simulink model "drones_simulation"  (R2025b)
settings: Solver=ode4  StartTime=0.0  StopTime=t_sim  FixedStep=Ts  RelTol=1e-3
values from neighbouring files (symbols this model uses):
  adj_row_1 = Adj_mat(1,:)    [Parameters_scenarios.m]
  adj_row_2 = Adj_mat(2,:)    [Parameters_scenarios.m]
  adj_row_3 = Adj_mat(3,:)    [Parameters_scenarios.m]
  adj_row_4 = Adj_mat(4,:)    [Parameters_scenarios.m]
  gamma1 = 8.0    (= 8)    [Parameters_scenarios.m]
  gamma2 = 8.0    (= 8)    [Parameters_scenarios.m]
  goal_tolerance = 0.05    [Parameters_scenarios.m]
  Ib = diag([Jxx, Jyy, Jzz])    [Parameters_scenarios.m]
  Kd = 2.5    [Parameters_scenarios.m]
  Kp = 1.2    [Parameters_scenarios.m]
  mass = 0.032    [Parameters_scenarios.m]
  max_acc = 2.5    [Parameters_scenarios.m]
  max_vel = 1.2 * (dist_total / desired_flight_time)    [Parameters_scenarios.m]
  Rc = 2.0    (= 2)    [Parameters_scenarios.m]
  Rs = Rs_safe    (= 0.15)    [Parameters_scenarios.m]
  Rs_obs = radius_robots + radii_obstacles + margin    (= 0.95)    [Parameters_scenarios.m]
  v0_1 = v0(1,:)'    [Parameters_scenarios.m]
  v0_2 = v0(2,:)'    [Parameters_scenarios.m]
  v0_3 = v0(3,:)'    [Parameters_scenarios.m]
  v0_4 = v0(4,:)'    [Parameters_scenarios.m]
  x0_1 = x0(1,:)'    [Parameters_scenarios.m]
  x0_2 = x0(2,:)'    [Parameters_scenarios.m]
  x0_3 = x0(3,:)'    [Parameters_scenarios.m]
  x0_4 = x0(4,:)'    [Parameters_scenarios.m]
  x_objects = [0.0 ... (first row only)    [Parameters_scenarios.m]
  xg_1 = xg(1,:)'    [Parameters_scenarios.m]
  xg_2 = xg(2,:)'    [Parameters_scenarios.m]
  xg_3 = xg(3,:)'    [Parameters_scenarios.m]
  xg_4 = xg(4,:)'    [Parameters_scenarios.m]
  xg_vec = reshape(xg', [], 1)    [Parameters_scenarios.m]
libraries: robotcorelib x4
(part 2 of 3)

== matlab function drones_simulation/Safety_and_connectivity_Drone_4/MATLAB Function10 ==
  data: x_i input; v_i input; u_safe output; x_neighbors input; v_neighbors input; u_gtg input; gamma1 input; gamma2 input; Rs input; x_obs input; Rs_obs input; x_comm input; v_comm input; Rc input; max_acc input
function u_safe = QPsafety_i(x_i, v_i, x_neighbors, v_neighbors, u_gtg, ...
                             gamma1, gamma2, Rs, x_obs, Rs_obs, ...
                             x_comm, v_comm, Rc, max_acc)
%QPsafety_i  Filtra un comando nominale u_gtg con un QP + vincoli CBF/HOCBF.
%
% IDEA:
%   - Variabile ottimizzata: u (accelerazione 3D).
%   - Obiettivo: restare il più vicino possibile al comando nominale u_gtg.
%   - Vincoli: evitare ostacoli, evitare collisioni con vicini, mantenere connettività,
%              e non scendere sotto una quota minima (pavimento virtuale).
%
% FORMA QP (quadprog):
%   min_u   1/2 u' H u + f' u
%   s.t.    A u <= b -> vincoli per mantenere distanze e connettività
%           lb <= u <=  -> vincolo per non superare i limiti di
%           accelerazione
%
% 
%   I vincoli CBF usano una forma tipo "relative degree 2":
%       h_ddot + gamma1*h_dot + gamma2*h >= 0
%   che diventa un vincolo lineare in u (quindi compatibile con quadprog).

    %% (0) Dimensione del problema
    n_dims = 3;   % accelerazione 3D [ux; uy; uz]

    %% (1) Output di default
    % Se non serve filtrare o il QP non trova soluzione, almeno ritorniamo qualcosa.
    u_safe = u_gtg;

    %% (2) Constraints sull'accelerazione
    lb = -max_acc * ones(n_dims, 1);
    ub =  max_acc * ones(n_dims, 1);

    %% (3) Costo del QP: minimizza ||u - u_gtg||^2
    % quadprog minimizza: 1/2 u'Hu + f'u
    % Con H=2I e f=-2u_gtg, si ottiene (a costante vicina):
    %    1/2 u'(2I)u + (-2u_gtg)'u = u'u - 2u_gtg'u  ~ ||u-u_gtg||^2
    H_qp = 2 * eye(n_dims);
    f_qp = -2 * u_gtg;

    %% (4) Matrici vincoli lineari (si riempiono aggiungendo righe)
    % Ogni ostacolo/vicino genera un vincolo lineare del tipo: a^T u <= b
    A = zeros(0, n_dims);
    b = zeros(0, 1);

    %% (5) VINCOLI 1: Ostacoli statici (evitamento)
    % Barriera: h = ||p - p_obs||^2 - R^2 >= 0  (stai FUORI dalla sfera di raggio R)
    % Con doppio integratore: h_ddot = LfLfh + LgLfh*u
    % Vincolo HOCBF: h_ddot + gamma1*h_dot + gamma2*h >= 0
    n_obs = size(x_obs, 2);

    for k = 1:n_obs
        p_o = x_obs(:, k);      % posizione ostacolo k
        R_o = Rs_obs(k);        % raggio di sicurezza ostacolo k

        rel_p = x_i - p_o;      % posizione relativa
        rel_v = v_i;            % ostacolo fermo => v_rel = v_i

        dist_sq = norm(rel_p)^2;
        h      = dist_sq - R_o^2;
        h_dot  = 2 * rel_p' * rel_v;

        % Per h = ||rel_p||^2 - R^2:
        % LgLfh = 2*rel_p' (coefficiente davanti a u)
        % LfLfh = 2*||rel_v||^2 (termine noto, non dipende da u)
        LgLfh = 2 * rel_p';
        LfLfh = 2 * (rel_v' * rel_v);

        % quadprog vuole A*u <= b.
        % Dalla forma HOCBF si arriva a:  -(LgLfh) * u <= LfLfh + gamma1*h_dot + gamma2*h
        A = [A; -LgLfh];
        b = [b; (LfLfh + gamma1*h_dot + gamma2*h)];
    end

    %% (6) VINCOLI 2: Vicini (anti-collisione inter-agente)
    % Stesso tipo di barriera degli ostacoli, ma con posizione/velocità relative:
    %   h = ||p_i - p_j||^2 - Rs^2 >= 0  (distanza minima Rs)
    valid_cols = ~isnan(x_neighbors(1,:));
    n_max_neighbors = size(x_neighbors, 2);

    for k = 1:n_max_neighbors
        if valid_cols(k)
            p_j = x_neighbors(:, k);
            v_j = v_neighbors(:, k);

            rel_p = x_i - p_j;
            rel_v = v_i - v_j;

            dist_sq = norm(rel_p)^2;
            h      = dist_sq - Rs^2;
            h_dot  = 2 * rel_p' * rel_v;

            LgLfh = 2 * rel_p';
            LfLfh = 2 * (rel_v' * rel_v);

            A = [A; -LgLfh];
            b = [b; (LfLfh + gamma1*h_dot + gamma2*h)];
        end
    end

    %% (7) VINCOLI 3: Connettività / coesione (non allontanarsi oltre Rc)
    % Qui la barriera è "invertita" (stai DENTRO):
    %   h_c = Rc^2 - ||p_i - p_c||^2 >= 0  =>  ||p_i - p_c|| <= Rc
    valid_cols_comm = ~isnan(x_comm(1,:));
    n_max_comm = size(x_comm, 2);

    for k = 1:n_max_comm
        if valid_cols_comm(k)
            p_c = x_comm(:, k);
            v_c = v_comm(:, k);

            rel_p = x_i - p_c;
            rel_v = v_i - v_c;

            dist_sq = norm(rel_p)^2;

            h_c     = Rc^2 - dist_sq;
            h_dot_c = -2 * rel_p' * rel_v;

            % Segni diversi rispetto al caso "stai fuori":
            LgLfh_c = -2 * rel_p';
            LfLfh_c = -2 * (rel_v' * rel_v);

            % Anche qui si porta tutto in A*u <= b:
            A = [A; -LgLfh_c];
            b = [b; (LfLfh_c + gamma1*h_dot_c + gamma2*h_c)];
        end
    end

    %% (8) VINCOLO 4: Pavimento virtuale (z >= z_limit)
    % Barriera: h = z - z_limit >= 0
    % Con doppio integratore: h_dot = v_z, h_ddot = u_z
    z_limit = 0.1;

    z_pos = x_i(3);
    z_vel = v_i(3);

    h_floor     = z_pos - z_limit;
    h_dot_floor = z_vel;

    % Seleziona solo la componente u_z:
    LgLfh_floor = [0, 0, 1];
    LfLfh_floor = 0;

    % Vincolo: u_z + gamma1*v_z + gamma2*(z-z_limit) >= 0
    % => -u_z <= gamma1*v_z + gamma2*h_floor
    A = [A; -LgLfh_floor];   % [0 0 -1]
    b = [b; (LfLfh_floor + gamma1*h_dot_floor + gamma2*h_floor)];

    %% (9) Risoluzione del QP
    % Se non ci sono vincoli, restituisci direttamente u_gtg.
    if isempty(A)
        u_safe = u_gtg;
        return;
    end

    options = optimoptions('quadprog', ...
        'Algorithm', 'active-set', ...
        'Display', 'off');

    % Punto iniziale per il solver (warm start semplice)
    u0 = zeros(n_dims, 1);

    % Risolvi:
    [u_opt, ~, exitflag] = quadprog(H_qp, f_qp, A, b, [], [], lb, ub, u0, options);

    %% (10) Scelta finale dell'azione
    if exitflag == 1
        % Soluzione trovata: comando sicuro
        u_safe = u_opt;
    else
        % QP infeasible / non risolto: fallback conservativo (frenata)
        % u = -k*v riduce la velocità rapidamente
        u_safe = -2.0 * v_i;
    end
end

== matlab function drones_simulation/Safety_and_connectivity_Drone_3/MATLAB Function11 ==
  data: x_neighbors output; x_i input; x_all input; v_all input; Rs input; v_neighbors output
function [x_neighbors, v_neighbors] = select_neighbors_i(x_i, x_all, v_all, Rs)
%Funzione usata per selezionare i vicini entro un raggio Rs dal robot i.
%
% SCOPO:
%   Dato lo stato del robot corrente (posizione x_i) e lo stato di tutti i robot
%   (x_all, v_all impacchettati in un unico vettore), questa funzione:
%   - scorre tutti i robot j
%   - scarta se stesso
%   - calcola la distanza tra i e j
%   - se j è entro Rs, lo inserisce nella lista dei vicini.
%
% INPUT:
%   x_i   : [3x1] posizione del robot corrente (p_i)
%   x_all : [3N x 1] posizioni di tutti i robot impacchettate
%           (x1;y1;z1; x2;y2;z2; ... ; xN;yN;zN)
%   v_all : [3N x 1] velocità di tutti i robot impacchettate
%           (vx1;vy1;vz1; vx2;vy2;vz2; ... )
%   Rs    : raggio di sicurezza
%
% OUTPUT:
%   x_neighbors : [3 x (N-1)] posizioni dei robot vicini trovati
%   v_neighbors : [3 x (N-1)] velocità dei robot vicini trovati
%   (Le colonne non usate restano NaN.)

    %% Parametri base
    n_dims   = 3;                          % dimensione spazio (x,y,z)
    n_robots = length(x_all) / n_dims;     % numero totale di robot N

    %% Preallocazione output con nan
    x_neighbors = nan(n_dims, n_robots-1);
    v_neighbors = nan(n_dims, n_robots-1);

    %% Contatore vicini trovati e raggio al quadrato
    count = 0;
    r_sq  = Rs^2;

    %% Scorri tutti i robot e seleziona quelli entro Rs
    for j = 1:n_robots

        %si estrae posizione e velocità del robot j dal vettore
        %impacchettato - INDICI
        idx_start = (j-1)*n_dims + 1;
        idx_end   = j*n_dims;

        p_j = x_all(idx_start : idx_end);  % [3x1] posizione robot j
        v_j = v_all(idx_start : idx_end);  % [3x1] velocità robot j

        % Si esclude il robot corrente 
        if norm(x_i - p_j) < 1e-6
            continue;
        end

        % Calcola la distanza al quadrato tra robot i e robot j
        dist_sq = sum((x_i - p_j).^2);

        % Se il robot j è entro Rs, aggiungilo alla lista dei vicini
        if dist_sq <= r_sq
            count = count + 1;

            x_neighbors(:, count) = p_j;
            v_neighbors(:, count) = v_j;
        end
    end

    % Al termine:
    % - Le prime "count" colonne contengono i vicini effettivi.
    % - Le colonne restanti rimangono NaN.
end

== matlab function drones_simulation/Safety_and_connectivity_Drone_4/MATLAB Function12 ==
  data: x_neighbors output; x_i input; x_all input; v_all input; Rs input; v_neighbors output
function [x_neighbors, v_neighbors] = select_neighbors_i(x_i, x_all, v_all, Rs)
%Funzione usata per selezionare i vicini entro un raggio Rs dal robot i.
%
% SCOPO:
%   Dato lo stato del robot corrente (posizione x_i) e lo stato di tutti i robot
%   (x_all, v_all impacchettati in un unico vettore), questa funzione:
%   - scorre tutti i robot j
%   - scarta se stesso
%   - calcola la distanza tra i e j
%   - se j è entro Rs, lo inserisce nella lista dei vicini.
%
% INPUT:
%   x_i   : [3x1] posizione del robot corrente (p_i)
%   x_all : [3N x 1] posizioni di tutti i robot impacchettate
%           (x1;y1;z1; x2;y2;z2; ... ; xN;yN;zN)
%   v_all : [3N x 1] velocità di tutti i robot impacchettate
%           (vx1;vy1;vz1; vx2;vy2;vz2; ... )
%   Rs    : raggio di sicurezza
%
% OUTPUT:
%   x_neighbors : [3 x (N-1)] posizioni dei robot vicini trovati
%   v_neighbors : [3 x (N-1)] velocità dei robot vicini trovati
%   (Le colonne non usate restano NaN.)

    %% Parametri base
    n_dims   = 3;                          % dimensione spazio (x,y,z)
    n_robots = length(x_all) / n_dims;     % numero totale di robot N

    %% Preallocazione output con nan
    x_neighbors = nan(n_dims, n_robots-1);
    v_neighbors = nan(n_dims, n_robots-1);

    %% Contatore vicini trovati e raggio al quadrato
    count = 0;
    r_sq  = Rs^2;

    %% Scorri tutti i robot e seleziona quelli entro Rs
    for j = 1:n_robots

        %si estrae posizione e velocità del robot j dal vettore
        %impacchettato - INDICI
        idx_start = (j-1)*n_dims + 1;
        idx_end   = j*n_dims;

        p_j = x_all(idx_start : idx_end);  % [3x1] posizione robot j
        v_j = v_all(idx_start : idx_end);  % [3x1] velocità robot j

        % Si esclude il robot corrente 
        if norm(x_i - p_j) < 1e-6
            continue;
        end

        % Calcola la distanza al quadrato tra robot i e robot j
        dist_sq = sum((x_i - p_j).^2);

        % Se il robot j è entro Rs, aggiungilo alla lista dei vicini
        if dist_sq <= r_sq
            count = count + 1;

            x_neighbors(:, count) = p_j;
            v_neighbors(:, count) = v_j;
        end
    end

    % Al termine:
    % - Le prime "count" colonne contengono i vicini effettivi.
    % - Le colonne restanti rimangono NaN.
end

== matlab function drones_simulation/MATLAB Function13 ==
  data: x_robot input; h_obs_vec output; x_objects input; Rs_objects input
function h_obs_vec = h_obs_checker(x_robot, x_objects, Rs_objects)
    % Calcola le dimensioni in base agli ostacoli
    n_dims = size(x_objects, 1); 
    
    % Numero di robot
    n_robots = length(x_robot) / n_dims;
    
    n_obs = size(x_objects, 2);
    h_obs_vec = zeros(n_robots * n_obs, 1); 
    
    k = 0;
    
    for i = 1:n_robots
   
  
        idx_start = (i-1)*n_dims + 1;
        idx_end   = i*n_dims;
        
        xi = x_robot(idx_start : idx_end); % Estrae vettore 3x1
        
        for o = 1:n_obs
            x_obs = x_objects(:, o); % Vettore 3x1
            Rs_o = Rs_objects(o);
            
            
            d2 = norm(xi - x_obs)^2;
            
            h = d2 - Rs_o^2;
            
            k = k + 1;
            h_obs_vec(k) = h;
        end
    end
end

== matlab function drones_simulation/Safety_and_connectivity_Drone_1/MATLAB Function14 ==
  data: x_comm output; x_all input; v_all input; adj_row input; my_id input; v_comm output
function [x_comm, v_comm] = select_comm_neighbors_i(x_all, v_all, adj_row, my_id)
% Questa funzione viene usata per poter trovare posizioni e velocità dei
% vicini di ogni singolo drone sulla base della matrice di connettività 
% Se due droni sono connessi, allora la matrice di connettività è pari a 1
% e allora si prendono x e v

    % INPUT:
    % x_all, v_all : [12x1] Stato di tutti i robot (posizione e velocità)
    % adj_row      : [1x4] Riga della matrice di adiacenza (es. [0 1 0 1])
    % my_id        : [1] ID del robot corrente (1, 2, 3 o 4)
    
    % OUTPUT:
    % x_comm_neigh : [3 x N_max] Posizioni vicini connessi
    % v_comm_neigh : [3 x N_max] Velocità vicini connessi

    n_dims = 3;
    max_neighbors = 3; % Numero massimo di connessioni previste
    
    % Inizializza con NaN
    x_comm = nan(n_dims, max_neighbors);
    v_comm = nan(n_dims, max_neighbors);
    
    n_robots = length(x_all) / n_dims;
    count = 0;
    
    for j = 1:n_robots
        % Se c'è un '1' nella matrice di adiacenza e non sono io 
        if j ~= my_id && adj_row(j) == 1
            count = count + 1;
            
            if count <= max_neighbors
                % Indici per estrarre vettori 3D
                k_start = (j-1)*n_dims + 1;
                k_end   = j*n_dims;
                
                % Estrai Posizione e Velocità
                x_comm(:, count) = x_all(k_start : k_end);
                v_comm(:, count) = v_all(k_start : k_end);
            end
        end
    end
end

== matlab function drones_simulation/Safety_and_connectivity_Drone_2/MATLAB Function15 ==
  data: x_comm output; x_all input; v_all input; adj_row input; my_id input; v_comm output
function [x_comm, v_comm] = select_comm_neighbors_i(x_all, v_all, adj_row, my_id)
% Questa funzione viene usata per poter trovare posizioni e velocità dei
% vicini di ogni singolo drone sulla base della matrice di connettività 
% Se due droni sono connessi, allora la matrice di connettività è pari a 1
% e allora si prendono x e v

    % INPUT:
    % x_all, v_all : [12x1] Stato di tutti i robot (posizione e velocità)
    % adj_row      : [1x4] Riga della matrice di adiacenza (es. [0 1 0 1])
    % my_id        : [1] ID del robot corrente (1, 2, 3 o 4)
    
    % OUTPUT:
    % x_comm_neigh : [3 x N_max] Posizioni vicini connessi
    % v_comm_neigh : [3 x N_max] Velocità vicini connessi

    n_dims = 3;
    max_neighbors = 3; % Numero massimo di connessioni previste
    
    % Inizializza con NaN
    x_comm = nan(n_dims, max_neighbors);
    v_comm = nan(n_dims, max_neighbors);
    
    n_robots = length(x_all) / n_dims;
    count = 0;
    
    for j = 1:n_robots
        % Se c'è un '1' nella matrice di adiacenza e non sono io 
        if j ~= my_id && adj_row(j) == 1
            count = count + 1;
            
            if count <= max_neighbors
                % Indici per estrarre vettori 3D
                k_start = (j-1)*n_dims + 1;
                k_end   = j*n_dims;
                
                % Estrai Posizione e Velocità
                x_comm(:, count) = x_all(k_start : k_end);
                v_comm(:, count) = v_all(k_start : k_end);
            end
        end
    end
end

== matlab function drones_simulation/Safety_and_connectivity_Drone_3/MATLAB Function16 ==
  data: x_comm output; x_all input; v_all input; adj_row input; my_id input; v_comm output
function [x_comm, v_comm] = select_comm_neighbors_i(x_all, v_all, adj_row, my_id)
% Questa funzione viene usata per poter trovare posizioni e velocità dei
% vicini di ogni singolo drone sulla base della matrice di connettività 
% Se due droni sono connessi, allora la matrice di connettività è pari a 1
% e allora si prendono x e v

    % INPUT:
    % x_all, v_all : [12x1] Stato di tutti i robot (posizione e velocità)
    % adj_row      : [1x4] Riga della matrice di adiacenza (es. [0 1 0 1])
    % my_id        : [1] ID del robot corrente (1, 2, 3 o 4)
    
    % OUTPUT:
    % x_comm_neigh : [3 x N_max] Posizioni vicini connessi
    % v_comm_neigh : [3 x N_max] Velocità vicini connessi

    n_dims = 3;
    max_neighbors = 3; % Numero massimo di connessioni previste
    
    % Inizializza con NaN
    x_comm = nan(n_dims, max_neighbors);
    v_comm = nan(n_dims, max_neighbors);
    
    n_robots = length(x_all) / n_dims;
    count = 0;
    
    for j = 1:n_robots
        % Se c'è un '1' nella matrice di adiacenza e non sono io 
        if j ~= my_id && adj_row(j) == 1
            count = count + 1;
            
            if count <= max_neighbors
                % Indici per estrarre vettori 3D
                k_start = (j-1)*n_dims + 1;
                k_end   = j*n_dims;
                
                % Estrai Posizione e Velocità
                x_comm(:, count) = x_all(k_start : k_end);
                v_comm(:, count) = v_all(k_start : k_end);
            end
        end
    end
end

== matlab function drones_simulation/Safety_and_connectivity_Drone_1/MATLAB Function1 ==
  data: x_neighbors output; x_i input; x_all input; v_all input; Rs input; v_neighbors output
function [x_neighbors, v_neighbors] = select_neighbors_i(x_i, x_all, v_all, Rs)
%Funzione usata per selezionare i vicini entro un raggio Rs dal robot i.
%
% SCOPO:
%   Dato lo stato del robot corrente (posizione x_i) e lo stato di tutti i robot
%   (x_all, v_all impacchettati in un unico vettore), questa funzione:
%   - scorre tutti i robot j
%   - scarta se stesso
%   - calcola la distanza tra i e j
%   - se j è entro Rs, lo inserisce nella lista dei vicini.
%
% INPUT:
%   x_i   : [3x1] posizione del robot corrente (p_i)
%   x_all : [3N x 1] posizioni di tutti i robot impacchettate
%           (x1;y1;z1; x2;y2;z2; ... ; xN;yN;zN)
%   v_all : [3N x 1] velocità di tutti i robot impacchettate
%           (vx1;vy1;vz1; vx2;vy2;vz2; ... )
%   Rs    : raggio di sicurezza
%
% OUTPUT:
%   x_neighbors : [3 x (N-1)] posizioni dei robot vicini trovati
%   v_neighbors : [3 x (N-1)] velocità dei robot vicini trovati
%   (Le colonne non usate restano NaN.)

    %% Parametri base
    n_dims   = 3;                          % dimensione spazio (x,y,z)
    n_robots = length(x_all) / n_dims;     % numero totale di robot N

    %% Preallocazione output con nan
    x_neighbors = nan(n_dims, n_robots-1);
    v_neighbors = nan(n_dims, n_robots-1);

    %% Contatore vicini trovati e raggio al quadrato
    count = 0;
    r_sq  = Rs^2;

    %% Scorri tutti i robot e seleziona quelli entro Rs
    for j = 1:n_robots

        %si estrae posizione e velocità del robot j dal vettore
        %impacchettato - INDICI
        idx_start = (j-1)*n_dims + 1;
        idx_end   = j*n_dims;

        p_j = x_all(idx_start : idx_end);  % [3x1] posizione robot j
        v_j = v_all(idx_start : idx_end);  % [3x1] velocità robot j

        % Si esclude il robot corrente 
        if norm(x_i - p_j) < 1e-6
            continue;
        end

        % Calcola la distanza al quadrato tra robot i e robot j
        dist_sq = sum((x_i - p_j).^2);

        % Se il robot j è entro Rs, aggiungilo alla lista dei vicini
        if dist_sq <= r_sq
            count = count + 1;

            x_neighbors(:, count) = p_j;
            v_neighbors(:, count) = v_j;
        end
    end

    % Al termine:
    % - Le prime "count" colonne contengono i vicini effettivi.
    % - Le colonne restanti rimangono NaN.
end

== matlab function drones_simulation/Safety_and_connectivity_Drone_4/MATLAB Function17 ==
  data: x_comm output; x_all input; v_all input; adj_row input; my_id input; v_comm output
function [x_comm, v_comm] = select_comm_neighbors_i(x_all, v_all, adj_row, my_id)
% Questa funzione viene usata per poter trovare posizioni e velocità dei
% vicini di ogni singolo drone sulla base della matrice di connettività 
% Se due droni sono connessi, allora la matrice di connettività è pari a 1
% e allora si prendono x e v

    % INPUT:
    % x_all, v_all : [12x1] Stato di tutti i robot (posizione e velocità)
    % adj_row      : [1x4] Riga della matrice di adiacenza (es. [0 1 0 1])
    % my_id        : [1] ID del robot corrente (1, 2, 3 o 4)
    
    % OUTPUT:
    % x_comm_neigh : [3 x N_max] Posizioni vicini connessi
    % v_comm_neigh : [3 x N_max] Velocità vicini connessi

    n_dims = 3;
    max_neighbors = 3; % Numero massimo di connessioni previste
    
    % Inizializza con NaN
    x_comm = nan(n_dims, max_neighbors);
    v_comm = nan(n_dims, max_neighbors);
    
    n_robots = length(x_all) / n_dims;
    count = 0;
    
    for j = 1:n_robots
        % Se c'è un '1' nella matrice di adiacenza e non sono io 
        if j ~= my_id && adj_row(j) == 1
            count = count + 1;
            
            if count <= max_neighbors
                % Indici per estrarre vettori 3D
                k_start = (j-1)*n_dims + 1;
                k_end   = j*n_dims;
                
                % Estrai Posizione e Velocità
                x_comm(:, count) = x_all(k_start : k_end);
                v_comm(:, count) = v_all(k_start : k_end);
            end
        end
    end
end

== matlab function drones_simulation/Subsystem_Drone_1/MATLAB Function ==
  data: u_safe input; Thrust output; psi_current input; m input; Phi_ref output; Theta_ref output
function [Thrust, Phi_ref, Theta_ref] = Accel_to_Attitude(u_safe, psi_current, m)
    % INPUT: u_safe [ax; ay; az], psi_current [rad], m [kg]
    g = 9.81;

    % THRUST
    % Calcoliamo la spinta necessaria per contrastare la gravità e accelerare
    acc_total_global = u_safe + [0; 0; g];
    raw_thrust = m * norm(acc_total_global);

    % Saturazione Thrust 
    max_thrust = m * g * 2.0; 
    Thrust = min(raw_thrust, max_thrust);

    % Rotazione Vettore Accelerazione (Global -> Body)
    ax_global = u_safe(1);
    ay_global = u_safe(2);

    % Proiettiamo la richiesta globale nel frame locale del drone ruotato di Yaw
    acc_body_x =  cos(psi_current) * ax_global + sin(psi_current) * ay_global;
    acc_body_y = -sin(psi_current) * ax_global + cos(psi_current) * ay_global;

    % CALCOLO DEGLI ANGOLI

    % PITCH (Theta):
    % Per andare AVANTI (+X), il drone deve abbassare il naso.
    % Abbassare il naso corrisponde a un angolo NEGATIVO.
    Theta_ref = +acc_body_x / g;  

    % ROLL (Phi):
    % Per andare a SINISTRA (+Y in body frame standard), serve un Roll NEGATIVO.
    % (Regola della mano destra: pollice su X, dita da Y a Z -> rotazione neg verso Y)
    Phi_ref   = -acc_body_y / g;

    % Saturazione Angoli 
    % Limitiamo l'inclinazione per mantenere valida l'approssimazione lineare
    max_angle = 0.52; % circa 30 gradi
    Theta_ref = max(min(Theta_ref, max_angle), -max_angle);
    Phi_ref   = max(min(Phi_ref, max_angle), -max_angle);
end

== matlab function drones_simulation/Subsystem_Drone_1/MATLAB Function1 ==
  data: Phi_ref input; Torques output; Theta_ref input; Psi_ref input; Phi input; Theta input; Psi input; p input; q input; r input
function Torques  = Attitude_Controller(Phi_ref, Theta_ref, Psi_ref, Phi, Theta, Psi, p, q, r)
    % INPUT:
    % *_ref: Angoli desiderati
    % Phi, Theta, Psi: Angoli attuali
    % p, q, r: Velocità angolari attuali
    
    % OUTPUT:
    % Torques: [3x1] Momenti [Tau_x; Tau_y; Tau_z]
    
    % GUADAGNI (piccoli dato che il drone è piccolo    
    % Roll (Phi)
    kp_phi = 0.05;   
    kd_phi = 0.0015;
    
    % Pitch (Theta)
    kp_theta = 0.05; 
    kd_theta = 0.0015;
    
    % Yaw (Psi) 
    kp_psi = 0.05;    
    kd_psi = 0.0015; 
    
    % CALCOLO ERRORI 
    e_phi   = Phi_ref - Phi;
    e_theta = Theta_ref - Theta;
    e_psi   = Psi_ref - Psi;
    
    % Gestione rapida discontinuità Yaw (Wrap to Pi) - forzatura tra -pi e
    % pi
    while e_psi > pi,  e_psi = e_psi - 2*pi; end
    while e_psi < -pi, e_psi = e_psi + 2*pi; end
    
    % CALCOLO MOMENTI (PD Control)
    tau_x = kp_phi   * e_phi   - kd_phi   * p;
    tau_y = kp_theta * e_theta - kd_theta * q;
    tau_z = kp_psi   * e_psi   - kd_psi   * r;
    
    % SATURAZIONE FISICA
    % Un micro-drone non può dare più di ~5-10 mNm di coppia.
    % Questo blocco impedisce l'errore "Derivative not finite".
    max_torque = 0.005; % 5 milli-Newton-metri
    
    tau_x = max(min(tau_x, max_torque), -max_torque);
    tau_y = max(min(tau_y, max_torque), -max_torque);
    tau_z = max(min(tau_z, max_torque), -max_torque);
    
    Torques = [tau_x; tau_y; tau_z];
end

== matlab function drones_simulation/Subsystem_Drone_1/Quadrotor dynamics/MATLAB Function1 ==
  data: Rb_temp input; Rb output
function Rb = fcn(Rb_temp)
    [U,S,V] = svd(Rb_temp);
    sigma = det(U*V');
    S_ = diag([1 1 sigma]);

    Rb = U*S_*V';
end

== matlab function drones_simulation/Subsystem_Drone_1/Quadrotor dynamics/UAV dynamics ==
  data: uT input size=1; tau_b input size=3; lin_acc output size=3; Rb input size=[3,3]; omega_bb input size=3; dot_Rb output size=[3,3]; ang_acc output size=3; mass parameter size=1; Ib parameter size=[3,3]
function [lin_acc, dot_Rb, ang_acc] = fcn(uT,tau_b,Rb,omega_bb,mass, Ib)

    g_vec = [0; 0; -9.81];
    thrust_vec_body = [0; 0; 1]; 
    
    % Accelerazione Lineare
    % Somma forze: Gravità + Spinta (Ruotata nel frame globale)
    lin_acc = g_vec + (uT / mass) * Rb * thrust_vec_body;
    
    % Derivata della Matrice di Rotazione (Cinematica)
    % R_dot = R * skew(omega)
    dot_Rb = Rb * skew(omega_bb);
    
    % Accelerazione Angolare (Eulero)
    % J*w_dot + w x J*w = Tau  -->  w_dot = J_inv * (Tau - w x J*w)
    ang_acc = inv(Ib) * (tau_b - skew(omega_bb) * Ib * omega_bb);

end

function S = skew(v)
if(numel(v)~= 1)
S= [0 -v(3) v(2); 
    v(3) 0 -v(1);
    -v(2) v(1) 0];
else
S= zeros(3);
end
end

== matlab function drones_simulation/Subsystem_Drone_2/MATLAB Function ==
  data: u_safe input; Thrust output; psi_current input; m input; Phi_ref output; Theta_ref output
function [Thrust, Phi_ref, Theta_ref] = Accel_to_Attitude(u_safe, psi_current, m)
    % INPUT: u_safe [ax; ay; az], psi_current [rad], m [kg]
    g = 9.81;

    % --- 1. Thrust ---
    % Calcoliamo la spinta necessaria per contrastare la gravità e accelerare
    acc_total_global = u_safe + [0; 0; g];
    raw_thrust = m * norm(acc_total_global);

    % Saturazione Thrust (importante per non destabilizzare)
    max_thrust = m * g * 2.0; 
    Thrust = min(raw_thrust, max_thrust);

    % --- 2. Rotazione Vettore Accelerazione (Global -> Body) ---
    ax_global = u_safe(1);
    ay_global = u_safe(2);

    % Proiettiamo la richiesta globale nel frame locale del drone ruotato di Yaw
    acc_body_x =  cos(psi_current) * ax_global + sin(psi_current) * ay_global;
    acc_body_y = -sin(psi_current) * ax_global + cos(psi_current) * ay_global;

    % --- 3. CALCOLO ANGOLI (CORREZIONE CRITICA) ---

    % PITCH (Theta):
    % Per andare AVANTI (+X), il drone deve abbassare il naso.
    % Abbassare il naso corrisponde a un angolo NEGATIVO.
    Theta_ref = +acc_body_x / g;  % <--- SEGNO MENO (CORRETTO)

    % ROLL (Phi):
    % Per andare a SINISTRA (+Y in body frame standard), serve un Roll NEGATIVO.
    % (Regola della mano destra: pollice su X, dita da Y a Z -> rotazione neg verso Y)
    Phi_ref   = -acc_body_y / g;  % <--- SEGNO MENO (CORRETTO)

    % --- 4. Saturazione Angoli ---
    % Limitiamo l'inclinazione per mantenere valida l'approssimazione lineare
    max_angle = 0.52; % circa 30 gradi
    Theta_ref = max(min(Theta_ref, max_angle), -max_angle);
    Phi_ref   = max(min(Phi_ref, max_angle), -max_angle);
end

== matlab function drones_simulation/Subsystem_Drone_2/MATLAB Function1 ==
  data: Phi_ref input; Torques output; Theta_ref input; Psi_ref input; Phi input; Theta input; Psi input; p input; q input; r input
function Torques  = Attitude_Controller(Phi_ref, Theta_ref, Psi_ref, Phi, Theta, Psi, p, q, r)
    % INPUT:
    % *_ref: Angoli desiderati
    % Phi, Theta, Psi: Angoli attuali
    % p, q, r: Velocità angolari attuali
    
    % OUTPUT:
    % Torques: [3x1] Momenti [Tau_x; Tau_y; Tau_z]
    
    % --- TUNING PID (Micro-Drone Crazyflie) ---
    % Inerzia approx 1.5e-5. I gains devono essere piccolissimi!
    
    % Roll (Phi) - Risposta veloce ma non esplosiva
    kp_phi = 0.05;   
    kd_phi = 0.0015;
    
    % Pitch (Theta)
    kp_theta = 0.05; 
    kd_theta = 0.0015;
    
    % Yaw (Psi) - Lo yaw è di solito più lento
    kp_psi = 0.05;    
    kd_psi = 0.0015; 
    
    % --- CALCOLO ERRORI ---
    e_phi   = Phi_ref - Phi;
    e_theta = Theta_ref - Theta;
    e_psi   = Psi_ref - Psi;
    
    % Gestione rapida discontinuità Yaw (Wrap to Pi)
    % Evita che se passi da 179 a -179 il drone faccia un giro completo
    while e_psi > pi,  e_psi = e_psi - 2*pi; end
    while e_psi < -pi, e_psi = e_psi + 2*pi; end
    
    % --- CALCOLO MOMENTI (PD Control) ---
    tau_x = kp_phi   * e_phi   - kd_phi   * p;
    tau_y = kp_theta * e_theta - kd_theta * q;
    tau_z = kp_psi   * e_psi   - kd_psi   * r;
    
    % --- SATURAZIONE FISICA (SALVAVITA) ---
    % Un micro-drone non può dare più di ~5-10 mNm di coppia.
    % Questo blocco impedisce l'errore "Derivative not finite".
    max_torque = 0.005; % 5 milli-Newton-metri
    
    tau_x = max(min(tau_x, max_torque), -max_torque);
    tau_y = max(min(tau_y, max_torque), -max_torque);
    tau_z = max(min(tau_z, max_torque), -max_torque);
    
    Torques = [tau_x; tau_y; tau_z];
end

== matlab function drones_simulation/Subsystem_Drone_2/Quadrotor dynamics/MATLAB Function1 ==
  data: Rb_temp input; Rb output
function Rb = fcn(Rb_temp)
    [U,S,V] = svd(Rb_temp);
    sigma = det(U*V');
    S_ = diag([1 1 sigma]);

    Rb = U*S_*V';
end

== matlab function drones_simulation/Subsystem_Drone_2/Quadrotor dynamics/UAV dynamics ==
  data: uT input size=1; tau_b input size=3; lin_acc output size=3; Rb input size=[3,3]; omega_bb input size=3; dot_Rb output size=[3,3]; ang_acc output size=3; mass parameter size=1; Ib parameter size=[3,3]
function [lin_acc, dot_Rb, ang_acc] = fcn(uT,tau_b,Rb,omega_bb,mass, Ib)

    g_vec = [0; 0; -9.81];
    thrust_vec_body = [0; 0; 1]; 
    
    % Accelerazione Lineare
    % Somma forze: Gravità + Spinta (Ruotata nel frame globale)
    lin_acc = g_vec + (uT / mass) * Rb * thrust_vec_body;
    
    % Derivata della Matrice di Rotazione (Cinematica)
    % R_dot = R * skew(omega)
    dot_Rb = Rb * skew(omega_bb);
    
    % Accelerazione Angolare (Eulero)
    % J*w_dot + w x J*w = Tau  -->  w_dot = J_inv * (Tau - w x J*w)
    ang_acc = inv(Ib) * (tau_b - skew(omega_bb) * Ib * omega_bb);

end

function S = skew(v)
if(numel(v)~= 1)
S= [0 -v(3) v(2); 
    v(3) 0 -v(1);
    -v(2) v(1) 0];
else
S= zeros(3);
end
end

== matlab function drones_simulation/MATLAB Function ==
  data: x_robot input; h_vec output; Rs input
function h_vec = h_checker_global(x_robot, Rs)
    % x_robot: Vettore colonna con TUTTE le posizioni [x1;y1;z1; x2;y2;z2; ...]
    % Rs: Raggio di sicurezza (scalare)
    
    % --- CONFIGURAZIONE 3D ---
    n_dims = 3; 
    
    % Calcola numero robot in base alla lunghezza del vettore input
    n_robots = length(x_robot) / n_dims;
    
    % Calcola il numero di coppie uniche: n*(n-1)/2
    % Esempio 4 robot: 4*3/2 = 6 coppie
    num_pairs = n_robots * (n_robots - 1) / 2;
    
    h_vec = zeros(num_pairs, 1);
    
    k = 0;
    
    % Doppio ciclo per confrontare ogni robot con gli altri (senza ripetizioni)
    for i = 1:n_robots
        % Indici per estrarre il robot i (3D)
        idx_i_start = (i-1)*n_dims + 1;
        idx_i_end   = i*n_dims;
        
        p_i = x_robot(idx_i_start : idx_i_end);
        
        for j = (i+1):n_robots
            % Indici per estrarre il robot j (3D)
            idx_j_start = (j-1)*n_dims + 1;
            idx_j_end   = j*n_dims;
            
            p_j = x_robot(idx_j_start : idx_j_end);
            
            % Calcolo distanza euclidea al quadrato in 3D
            dist_sq = norm(p_i - p_j)^2;
            
            % Calcolo funzione barriera h
            val_h = dist_sq - Rs^2;
            
            k = k + 1;
            h_vec(k) = val_h;
        end
    end
end

== matlab function drones_simulation/Subsystem_Drone_3/MATLAB Function ==
  data: u_safe input; Thrust output; psi_current input; m input; Phi_ref output; Theta_ref output
function [Thrust, Phi_ref, Theta_ref] = Accel_to_Attitude(u_safe, psi_current, m)
    % INPUT: u_safe [ax; ay; az], psi_current [rad], m [kg]
    g = 9.81;

    % --- 1. Thrust ---
    % Calcoliamo la spinta necessaria per contrastare la gravità e accelerare
    acc_total_global = u_safe + [0; 0; g];
    raw_thrust = m * norm(acc_total_global);

    % Saturazione Thrust (importante per non destabilizzare)
    max_thrust = m * g * 2.0; 
    Thrust = min(raw_thrust, max_thrust);

    % --- 2. Rotazione Vettore Accelerazione (Global -> Body) ---
    ax_global = u_safe(1);
    ay_global = u_safe(2);

    % Proiettiamo la richiesta globale nel frame locale del drone ruotato di Yaw
    acc_body_x =  cos(psi_current) * ax_global + sin(psi_current) * ay_global;
    acc_body_y = -sin(psi_current) * ax_global + cos(psi_current) * ay_global;

    % --- 3. CALCOLO ANGOLI (CORREZIONE CRITICA) ---

    % PITCH (Theta):
    % Per andare AVANTI (+X), il drone deve abbassare il naso.
    % Abbassare il naso corrisponde a un angolo NEGATIVO.
    Theta_ref = +acc_body_x / g;  % <--- SEGNO MENO (CORRETTO)

    % ROLL (Phi):
    % Per andare a SINISTRA (+Y in body frame standard), serve un Roll NEGATIVO.
    % (Regola della mano destra: pollice su X, dita da Y a Z -> rotazione neg verso Y)
    Phi_ref   = -acc_body_y / g;  % <--- SEGNO MENO (CORRETTO)

    % --- 4. Saturazione Angoli ---
    % Limitiamo l'inclinazione per mantenere valida l'approssimazione lineare
    max_angle = 0.52; % circa 30 gradi
    Theta_ref = max(min(Theta_ref, max_angle), -max_angle);
    Phi_ref   = max(min(Phi_ref, max_angle), -max_angle);
end

== matlab function drones_simulation/Subsystem_Drone_3/MATLAB Function1 ==
  data: Phi_ref input; Torques output; Theta_ref input; Psi_ref input; Phi input; Theta input; Psi input; p input; q input; r input
function Torques  = Attitude_Controller(Phi_ref, Theta_ref, Psi_ref, Phi, Theta, Psi, p, q, r)
    % INPUT:
    % *_ref: Angoli desiderati
    % Phi, Theta, Psi: Angoli attuali
    % p, q, r: Velocità angolari attuali
    
    % OUTPUT:
    % Torques: [3x1] Momenti [Tau_x; Tau_y; Tau_z]
    
    % --- TUNING PID (Micro-Drone Crazyflie) ---
    % Inerzia approx 1.5e-5. I gains devono essere piccolissimi!
    
    % Roll (Phi) - Risposta veloce ma non esplosiva
    kp_phi = 0.05;   
    kd_phi = 0.0015;
    
    % Pitch (Theta)
    kp_theta = 0.05; 
    kd_theta = 0.0015;
    
    % Yaw (Psi) - Lo yaw è di solito più lento
    kp_psi = 0.05;    
    kd_psi = 0.0015; 
    
    % --- CALCOLO ERRORI ---
    e_phi   = Phi_ref - Phi;
    e_theta = Theta_ref - Theta;
    e_psi   = Psi_ref - Psi;
    
    % Gestione rapida discontinuità Yaw (Wrap to Pi)
    % Evita che se passi da 179 a -179 il drone faccia un giro completo
    while e_psi > pi,  e_psi = e_psi - 2*pi; end
    while e_psi < -pi, e_psi = e_psi + 2*pi; end
    
    % --- CALCOLO MOMENTI (PD Control) ---
    tau_x = kp_phi   * e_phi   - kd_phi   * p;
    tau_y = kp_theta * e_theta - kd_theta * q;
    tau_z = kp_psi   * e_psi   - kd_psi   * r;
    
    % --- SATURAZIONE FISICA (SALVAVITA) ---
    % Un micro-drone non può dare più di ~5-10 mNm di coppia.
    % Questo blocco impedisce l'errore "Derivative not finite".
    max_torque = 0.005; % 5 milli-Newton-metri
    
    tau_x = max(min(tau_x, max_torque), -max_torque);
    tau_y = max(min(tau_y, max_torque), -max_torque);
    tau_z = max(min(tau_z, max_torque), -max_torque);
    
    Torques = [tau_x; tau_y; tau_z];
end

== matlab function drones_simulation/Subsystem_Drone_3/Quadrotor dynamics/MATLAB Function1 ==
  data: Rb_temp input; Rb output
function Rb = fcn(Rb_temp)
    [U,S,V] = svd(Rb_temp);
    sigma = det(U*V');
    S_ = diag([1 1 sigma]);

    Rb = U*S_*V';
end

== matlab function drones_simulation/Subsystem_Drone_3/Quadrotor dynamics/UAV dynamics ==
  data: uT input size=1; tau_b input size=3; lin_acc output size=3; Rb input size=[3,3]; omega_bb input size=3; dot_Rb output size=[3,3]; ang_acc output size=3; mass parameter size=1; Ib parameter size=[3,3]
function [lin_acc, dot_Rb, ang_acc] = fcn(uT,tau_b,Rb,omega_bb,mass, Ib)

    g_vec = [0; 0; -9.81];
    thrust_vec_body = [0; 0; 1]; 
    
    % Accelerazione Lineare
    % Somma forze: Gravità + Spinta (Ruotata nel frame globale)
    lin_acc = g_vec + (uT / mass) * Rb * thrust_vec_body;
    
    % Derivata della Matrice di Rotazione (Cinematica)
    % R_dot = R * skew(omega)
    dot_Rb = Rb * skew(omega_bb);
    
    % Accelerazione Angolare (Eulero)
    % J*w_dot + w x J*w = Tau  -->  w_dot = J_inv * (Tau - w x J*w)
    ang_acc = inv(Ib) * (tau_b - skew(omega_bb) * Ib * omega_bb);

end

function S = skew(v)
if(numel(v)~= 1)
S= [0 -v(3) v(2); 
    v(3) 0 -v(1);
    -v(2) v(1) 0];
else
S= zeros(3);
end
end

== matlab function drones_simulation/Subsystem_Drone_4/MATLAB Function ==
  data: u_safe input; Thrust output; psi_current input; m input; Phi_ref output; Theta_ref output
function [Thrust, Phi_ref, Theta_ref] = Accel_to_Attitude(u_safe, psi_current, m)
    % INPUT: u_safe [ax; ay; az], psi_current [rad], m [kg]
    g = 9.81;

    % --- 1. Thrust ---
    % Calcoliamo la spinta necessaria per contrastare la gravità e accelerare
    acc_total_global = u_safe + [0; 0; g];
    raw_thrust = m * norm(acc_total_global);

    % Saturazione Thrust (importante per non destabilizzare)
    max_thrust = m * g * 2.0; 
    Thrust = min(raw_thrust, max_thrust);

    % --- 2. Rotazione Vettore Accelerazione (Global -> Body) ---
    ax_global = u_safe(1);
    ay_global = u_safe(2);

    % Proiettiamo la richiesta globale nel frame locale del drone ruotato di Yaw
    acc_body_x =  cos(psi_current) * ax_global + sin(psi_current) * ay_global;
    acc_body_y = -sin(psi_current) * ax_global + cos(psi_current) * ay_global;

    % --- 3. CALCOLO ANGOLI (CORREZIONE CRITICA) ---

    % PITCH (Theta):
    % Per andare AVANTI (+X), il drone deve abbassare il naso.
    % Abbassare il naso corrisponde a un angolo NEGATIVO.
    Theta_ref = +acc_body_x / g;  % <--- SEGNO MENO (CORRETTO)

    % ROLL (Phi):
    % Per andare a SINISTRA (+Y in body frame standard), serve un Roll NEGATIVO.
    % (Regola della mano destra: pollice su X, dita da Y a Z -> rotazione neg verso Y)
    Phi_ref   = -acc_body_y / g;  % <--- SEGNO MENO (CORRETTO)

    % --- 4. Saturazione Angoli ---
    % Limitiamo l'inclinazione per mantenere valida l'approssimazione lineare
    max_angle = 0.52; % circa 30 gradi
    Theta_ref = max(min(Theta_ref, max_angle), -max_angle);
    Phi_ref   = max(min(Phi_ref, max_angle), -max_angle);
end

== matlab function drones_simulation/Subsystem_Drone_4/MATLAB Function1 ==
  data: Phi_ref input; Torques output; Theta_ref input; Psi_ref input; Phi input; Theta input; Psi input; p input; q input; r input
function Torques  = Attitude_Controller(Phi_ref, Theta_ref, Psi_ref, Phi, Theta, Psi, p, q, r)
    % INPUT:
    % *_ref: Angoli desiderati
    % Phi, Theta, Psi: Angoli attuali
    % p, q, r: Velocità angolari attuali
    
    % OUTPUT:
    % Torques: [3x1] Momenti [Tau_x; Tau_y; Tau_z]
    
    % --- TUNING PID (Micro-Drone Crazyflie) ---
    % Inerzia approx 1.5e-5. I gains devono essere piccolissimi!
    
    % Roll (Phi) - Risposta veloce ma non esplosiva
    kp_phi = 0.05;   
    kd_phi = 0.0015;
    
    % Pitch (Theta)
    kp_theta = 0.05; 
    kd_theta = 0.0015;
    
    % Yaw (Psi) - Lo yaw è di solito più lento
    kp_psi = 0.05;    
    kd_psi = 0.0015; 
    
    % --- CALCOLO ERRORI ---
    e_phi   = Phi_ref - Phi;
    e_theta = Theta_ref - Theta;
    e_psi   = Psi_ref - Psi;
    
    % Gestione rapida discontinuità Yaw (Wrap to Pi)
    % Evita che se passi da 179 a -179 il drone faccia un giro completo
    while e_psi > pi,  e_psi = e_psi - 2*pi; end
    while e_psi < -pi, e_psi = e_psi + 2*pi; end
    
    % --- CALCOLO MOMENTI (PD Control) ---
    tau_x = kp_phi   * e_phi   - kd_phi   * p;
    tau_y = kp_theta * e_theta - kd_theta * q;
    tau_z = kp_psi   * e_psi   - kd_psi   * r;
    
    % --- SATURAZIONE FISICA (SALVAVITA) ---
    % Un micro-drone non può dare più di ~5-10 mNm di coppia.
    % Questo blocco impedisce l'errore "Derivative not finite".
    max_torque = 0.005; % 5 milli-Newton-metri
    
    tau_x = max(min(tau_x, max_torque), -max_torque);
    tau_y = max(min(tau_y, max_torque), -max_torque);
    tau_z = max(min(tau_z, max_torque), -max_torque);
    
    Torques = [tau_x; tau_y; tau_z];
end

== matlab function drones_simulation/Subsystem_Drone_4/Quadrotor dynamics/MATLAB Function1 ==
  data: Rb_temp input; Rb output
function Rb = fcn(Rb_temp)
    [U,S,V] = svd(Rb_temp);
    sigma = det(U*V');
    S_ = diag([1 1 sigma]);

    Rb = U*S_*V';
end

== matlab function drones_simulation/Safety_and_connectivity_Drone_2/MATLAB Function2 ==
  data: x_neighbors output; x_i input; x_all input; v_all input; Rs input; v_neighbors output
function [x_neighbors, v_neighbors] = select_neighbors_i(x_i, x_all, v_all, Rs)
%Funzione usata per selezionare i vicini entro un raggio Rs dal robot i.
%
% SCOPO:
%   Dato lo stato del robot corrente (posizione x_i) e lo stato di tutti i robot
%   (x_all, v_all impacchettati in un unico vettore), questa funzione:
%   - scorre tutti i robot j
%   - scarta se stesso
%   - calcola la distanza tra i e j
%   - se j è entro Rs, lo inserisce nella lista dei vicini.
%
% INPUT:
%   x_i   : [3x1] posizione del robot corrente (p_i)
%   x_all : [3N x 1] posizioni di tutti i robot impacchettate
%           (x1;y1;z1; x2;y2;z2; ... ; xN;yN;zN)
%   v_all : [3N x 1] velocità di tutti i robot impacchettate
%           (vx1;vy1;vz1; vx2;vy2;vz2; ... )
%   Rs    : raggio di sicurezza
%
% OUTPUT:
%   x_neighbors : [3 x (N-1)] posizioni dei robot vicini trovati
%   v_neighbors : [3 x (N-1)] velocità dei robot vicini trovati
%   (Le colonne non usate restano NaN.)

    %% Parametri base
    n_dims   = 3;                          % dimensione spazio (x,y,z)
    n_robots = length(x_all) / n_dims;     % numero totale di robot N

    %% Preallocazione output con nan
    x_neighbors = nan(n_dims, n_robots-1);
    v_neighbors = nan(n_dims, n_robots-1);

    %% Contatore vicini trovati e raggio al quadrato
    count = 0;
    r_sq  = Rs^2;

    %% Scorri tutti i robot e seleziona quelli entro Rs
    for j = 1:n_robots

        %si estrae posizione e velocità del robot j dal vettore
        %impacchettato - INDICI
        idx_start = (j-1)*n_dims + 1;
        idx_end   = j*n_dims;

        p_j = x_all(idx_start : idx_end);  % [3x1] posizione robot j
        v_j = v_all(idx_start : idx_end);  % [3x1] velocità robot j

        % Si esclude il robot corrente 
        if norm(x_i - p_j) < 1e-6
            continue;
        end

        % Calcola la distanza al quadrato tra robot i e robot j
        dist_sq = sum((x_i - p_j).^2);

        % Se il robot j è entro Rs, aggiungilo alla lista dei vicini
        if dist_sq <= r_sq
            count = count + 1;

            x_neighbors(:, count) = p_j;
            v_neighbors(:, count) = v_j;
        end
    end

    % Al termine:
    % - Le prime "count" colonne contengono i vicini effettivi.
    % - Le colonne restanti rimangono NaN.
end

== matlab function drones_simulation/Subsystem_Drone_4/Quadrotor dynamics/UAV dynamics ==
  data: uT input size=1; tau_b input size=3; lin_acc output size=3; Rb input size=[3,3]; omega_bb input size=3; dot_Rb output size=[3,3]; ang_acc output size=3; mass parameter size=1; Ib parameter size=[3,3]
function [lin_acc, dot_Rb, ang_acc] = fcn(uT,tau_b,Rb,omega_bb,mass, Ib)

    g_vec = [0; 0; -9.81];
    thrust_vec_body = [0; 0; 1]; 
    
    % Accelerazione Lineare
    % Somma forze: Gravità + Spinta (Ruotata nel frame globale)
    lin_acc = g_vec + (uT / mass) * Rb * thrust_vec_body;
    
    % Derivata della Matrice di Rotazione (Cinematica)
    % R_dot = R * skew(omega)
    dot_Rb = Rb * skew(omega_bb);
    
    % Accelerazione Angolare (Eulero)
    % J*w_dot + w x J*w = Tau  -->  w_dot = J_inv * (Tau - w x J*w)
    ang_acc = inv(Ib) * (tau_b - skew(omega_bb) * Ib * omega_bb);

end

function S = skew(v)
if(numel(v)~= 1)
S= [0 -v(3) v(2); 
    v(3) 0 -v(1);
    -v(2) v(1) 0];
else
S= zeros(3);
end
end

== matlab function drones_simulation/MATLAB Function18 ==
  data: x_all input; stop_sim output; xg_vec input; tol input; n_robots input
function stop_sim = Check_Stop_Condition(x_all, xg_vec, tol, n_robots)
% questa funzione serve per fermare la simulazione del momento in cui i
% robot hanno raggiunto i rispettivi goal entro una tollerance e ci restano
% un certo tempo
    % INPUT:
    % x_all: [3*N x 1] vettore con tutte le posizioni attuali
    % xg_vec: [3*N x 1] vettore con tutti i goal 
    % tol: scalare, distanza minima
    % n_robots: numero robot (es. 4)
    
    % OUTPUT:
    % stop_sim: booleano (1 = STOP, 0 = CONTINUA)
    
    persistent all_reached_count
    if isempty(all_reached_count)
        all_reached_count = 0;
    end
    
    stop_signal = true; % Assumiamo che abbiano finito tutti, poi verifichiamo
    
    for i = 1:n_robots
        % Estrai indici
        idx = (i-1)*3 + (1:3);
        
        p_curr = x_all(idx);
        p_goal = xg_vec(idx);
        
        % Calcola errore
        dist = norm(p_curr - p_goal);
        
        % Se ANCHE UNO SOLO è fuori tolleranza, non ci fermiamo
        if dist > tol
            stop_signal = false;
            break;
        end
    end
    
    % Aspettiamo che rimangano fermi sul goal per un po' 
    % per evitare che si fermi se uno passa per sbaglio sul goal veloce.
    if stop_signal
        all_reached_count = all_reached_count + 1;
    else
        all_reached_count = 0;
    end
    
    % Se tutti sono sul goal da almeno 0.1 secondi (100 step a 1kHz), STOP.
    if all_reached_count > 100 
        stop_sim = 1;
    else
        stop_sim = 0;
    end
end

== matlab function drones_simulation/MATLAB Function3 ==
  data: x_i input; v_i input; u_gtg output; xg_i input; Kp input; Kd input; max_acc input; max_vel input
function u_gtg = controller_generic(x_i, v_i, xg_i, Kp, Kd, max_acc, max_vel)

    % Errore posizione
    e_p = xg_i - x_i;
    
    % Velocità Desiderata (Proporzionale all'errore)
    % Il termine Kp * e_p è idealmente la velocità che vorremmo avere
    
    v_des = (Kp / Kd) * e_p; % velocità proporzionale all'errore di posizione
    
    % Saturazione della velocità desiderata 
    v_norm = norm(v_des);
    if v_norm > max_vel
        v_des = (v_des / v_norm) * max_vel;
    end
    
    % Controllo dove si insegue la velocità
    u_unclamped = Kd * (v_des - v_i); % equivalente a un PD classico u = Kp*ep - Kd*v
    
    % 4. Saturazione accelerazione 
    norm_u = norm(u_unclamped);
    if norm_u > max_acc
        u_gtg = (u_unclamped / norm_u) * max_acc;
    else
        u_gtg = u_unclamped;
    end
end

== matlab function drones_simulation/MATLAB Function4 ==
  data: x_i input; v_i input; u_gtg output; xg_i input; Kp input; Kd input; max_acc input; max_vel input
function u_gtg = controller_generic(x_i, v_i, xg_i, Kp, Kd, max_acc, max_vel)

    % Errore posizione
    e_p = xg_i - x_i;
    
    % Velocità Desiderata (Proporzionale all'errore)
    % Il termine Kp * e_p è idealmente la velocità che vorremmo avere
    
    v_des = (Kp / Kd) * e_p; % velocità proporzionale all'errore di posizione
    
    % Saturazione della velocità desiderata 
    v_norm = norm(v_des);
    if v_norm > max_vel
        v_des = (v_des / v_norm) * max_vel;
    end
    
    % Controllo dove si insegue la velocità
    u_unclamped = Kd * (v_des - v_i); % equivalente a un PD classico u = Kp*ep - Kd*v
    
    % 4. Saturazione accelerazione 
    norm_u = norm(u_unclamped);
    if norm_u > max_acc
        u_gtg = (u_unclamped / norm_u) * max_acc;
    else
        u_gtg = u_unclamped;
    end
end
